simulink model "lfc_3area"  (R2026a)
settings: Solver=ode4  StopTime=60  FixedStep=0.01
model workspace (MATLAB code in the model file):
  | % lfc_params_3area.m
  | % ------------------------------------------------------------------------
  | % Parameters for the THREE-area LFC Simulink model (lfc_3area.slx).
  | %
  | % Physical parameters come from Table I of:
  | %   Shangguan et al., "Detection and Defense Against Multi-Point False Data
  | %   Injection Attacks of Load Frequency Control in Smart Grid,"
  | %   IEEE Trans. Smart Grid, vol. 16, no. 5, pp. 4143-4154, Sep. 2025.
  | %
  | % Each area's dual turbine-governor "a/b" entries are collapsed into a
  | % single-machine equivalent by averaging, so the per-area single-state
  | % equations (1a)-(1c) apply exactly (same convention as the Python
  | % replication in ../lfc_fdi_replication/config.py).
  | %
  | % Units: p.u. on a 3000 MVA base, frequency deviation in Hz.
  | % ------------------------------------------------------------------------
  | 
  | % ---- Area 1 ----
  | Tg1 = 0.320;  Tt1 = 0.065;  R1 = 2.835;  M1 = 0.1500;  D1 = 0.0640;
  | beta1 = 0.4250;  Kp1 = 0.0554;  Ki1 = 0.2285;
  | 
  | % ---- Area 2 ----
  | Tg2 = 0.305;  Tt2 = 0.080;  R2 = 2.945;  M2 = 0.1875;  D2 = 0.0964;
  | beta2 = 0.3966;  Kp2 = 0.0475;  Ki2 = 0.1764;
  | 
  | % ---- Area 3 ----
  | Tg3 = 0.320;  Tt3 = 0.060;  R3 = 2.725;  M3 = 0.1440;  D3 = 0.0850;
  | beta3 = 0.3552;  Kp3 = 0.0444;  Ki3 = 0.1866;
  | 
  | % ---- Tie-line synchronizing coefficients (Table I) ----
  | T12 = 0.243;  T13 = 0.321;  T23 = 0.195;
  | 
  | % ---- HVDC link equivalents per tie (average of the two areas' Kdc/Tdc) ----
  | % Area gains: Kdc = [0.90 1.10 0.86], Tdc = [0.50 0.55 0.48]
  | Kdc12 = 1.00;   Tdc12 = 0.525;
  | Kdc13 = 0.88;   Tdc13 = 0.490;
  | Kdc23 = 0.98;   Tdc23 = 0.515;
  | 
  | % ---- Nonlinearities (Section IV-A) ----
  | gdb = 6e-4;     % governor dead-band half-width [p.u.]
  | grc = 0.05;     % generation rate constraint [p.u./s]
  | 
  | % ---- Load / RES step disturbances per area ----
  | Pd1_t = 1;  Pd1_mag = 0.02;      % 0.02 p.u. load step in area 1 at t = 1 s
  | Pd2_t = 1;  Pd2_mag = 0;
  | Pd3_t = 1;  Pd3_mag = 0;
  | Pres1_t = 1;  Pres1_mag = 0;
  | Pres2_t = 1;  Pres2_mag = 0;
  | Pres3_t = 1;  Pres3_mag = 0;
  | 
  | % ---- FDI attack settings (Section II-B), one injector per channel -------
  | % Channel signal:  A(t) = gate(t) * [ step + samp*sin(w*(t-t0)) + pulse_train ]
  | % gate(t) = 1 for t0 <= t <= t1, else 0.  Set all magnitudes to 0 => no attack.
  | atk_pw = 3;                        % pulse on/off width [s]
  | chans = {'df1','df2','df3','pt1','pt2','pt3'};
  | for c = 1:numel(chans)
  |     ch = chans{c};
  |     eval(sprintf(['atk_%s_t0 = 20; atk_%s_t1 = 40; atk_%s_step = 0; ' ...
  |         'atk_%s_samp = 0; atk_%s_w = 2; atk_%s_pulse = 0;'], ...
  |         ch, ch, ch, ch, ch, ch));
  | end
  | clear chans c ch
undefined symbols (not defined in the file): atk_df1_pulse, atk_df1_samp, atk_df1_step, atk_df1_t0, atk_df1_t1, atk_df1_w, atk_df2_pulse, atk_df2_samp, atk_df2_step, atk_df2_t0, atk_df2_t1, atk_df2_w, atk_df3_pulse, atk_df3_samp, atk_df3_step, atk_df3_t0, atk_df3_t1, atk_df3_w, atk_pt1_pulse, atk_pt1_samp, atk_pt1_step, atk_pt1_t0, atk_pt1_t1, atk_pt1_w, atk_pt2_pulse, atk_pt2_samp, atk_pt2_step, atk_pt2_t0, atk_pt2_t1, atk_pt2_w, atk_pt3_pulse, atk_pt3_samp, atk_pt3_step, atk_pt3_t0, atk_pt3_t1, atk_pt3_w
settings Model: Creator=gunnalakistagoud  LastModifiedBy=gunnalakistagoud

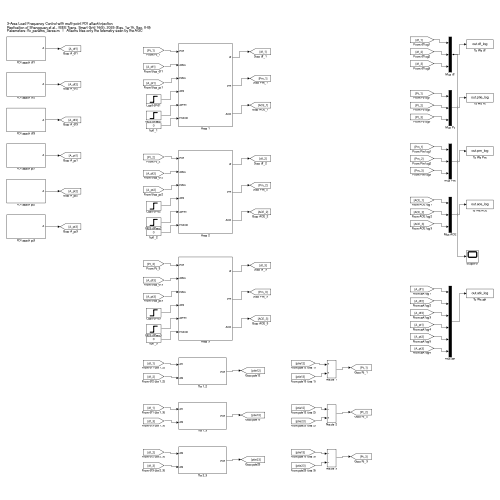
[thumbnail: Simulink's stored preview of the top-level diagram]
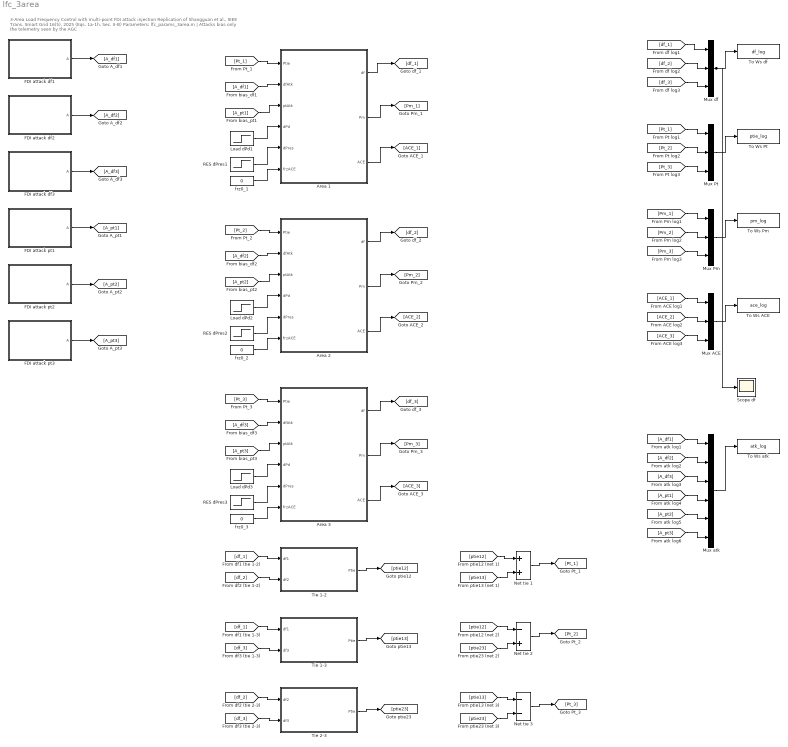
== system lfc_3area ==
  note: 3-Area Load Frequency Control with multi-point FDI attack injection
      | Replication of Shangguan et al., IEEE Trans. Smart Grid 16(5), 2025 (Eqs. 1a-1h, Sec. II-B)
      | Parameters: lfc_params_3area.m   |   Attacks bias only the telemetry seen by the AGC
  Area 1 : Subsystem
  Area 2 : Subsystem
  Area 3 : Subsystem
  FDI attack df1 : Subsystem
  FDI attack df2 : Subsystem
  FDI attack df3 : Subsystem
  FDI attack pt1 : Subsystem
  FDI attack pt2 : Subsystem
  FDI attack pt3 : Subsystem
  Load dPd1 : Step  Time=Pd1_t  FinalValue=Pd1_mag  SampleTime=0
  Load dPd2 : Step  Time=Pd2_t  FinalValue=Pd2_mag  SampleTime=0
  Load dPd3 : Step  Time=Pd3_t  FinalValue=Pd3_mag  SampleTime=0
  Mux ACE : Mux  Inputs=3
  Mux Pm : Mux  Inputs=3
  Mux Pt : Mux  Inputs=3
  Mux atk : Mux  Inputs=6
  Mux df : Mux  Inputs=3
  Net tie 1 : Sum
  Net tie 2 : Sum  Inputs=-+
  Net tie 3 : Sum  Inputs=--
  RES dPres1 : Step  Time=Pres1_t  FinalValue=Pres1_mag  SampleTime=0
  RES dPres2 : Step  Time=Pres2_t  FinalValue=Pres2_mag  SampleTime=0
  RES dPres3 : Step  Time=Pres3_t  FinalValue=Pres3_mag  SampleTime=0
  Scope df : Scope
  Tie 1-2 : Subsystem
  Tie 1-3 : Subsystem
  Tie 2-3 : Subsystem
  To Ws ACE : ToWorkspace  VariableName=ace_log  SaveFormat=Timeseries  SampleTime=-1
  To Ws Pm : ToWorkspace  VariableName=pm_log  SaveFormat=Timeseries  SampleTime=-1
  To Ws Pt : ToWorkspace  VariableName=ptie_log  SaveFormat=Timeseries  SampleTime=-1
  To Ws atk : ToWorkspace  VariableName=atk_log  SaveFormat=Timeseries  SampleTime=-1
  To Ws df : ToWorkspace  VariableName=df_log  SaveFormat=Timeseries  SampleTime=-1
  frz0_1 : Constant  Value=0
  frz0_2 : Constant  Value=0
  frz0_3 : Constant  Value=0
  wires:
  FDI attack df1/1(A) -> [A_df1]
  FDI attack df2/1(A) -> [A_df2]
  FDI attack df3/1(A) -> [A_df3]
  FDI attack pt1/1(A) -> [A_pt1]
  FDI attack pt2/1(A) -> [A_pt2]
  FDI attack pt3/1(A) -> [A_pt3]
  [Pt_1] -> Area 1/1(Ptie)
  [A_df1] -> Area 1/2(dfAtk)
  [A_pt1] -> Area 1/3(ptAtk)
  Load dPd1/1 -> Area 1/4(dPd)
  RES dPres1/1 -> Area 1/5(dPres)
  frz0_1/1 -> Area 1/6(frzACE)
  Area 1/1(df) -> [df_1]
  Area 1/2(Pm) -> [Pm_1]
  Area 1/3(ACE) -> [ACE_1]
  [Pt_2] -> Area 2/1(Ptie)
  [A_df2] -> Area 2/2(dfAtk)
  [A_pt2] -> Area 2/3(ptAtk)
  Load dPd2/1 -> Area 2/4(dPd)
  RES dPres2/1 -> Area 2/5(dPres)
  frz0_2/1 -> Area 2/6(frzACE)
  Area 2/1(df) -> [df_2]
  Area 2/2(Pm) -> [Pm_2]
  Area 2/3(ACE) -> [ACE_2]
  [Pt_3] -> Area 3/1(Ptie)
  [A_df3] -> Area 3/2(dfAtk)
  [A_pt3] -> Area 3/3(ptAtk)
  Load dPd3/1 -> Area 3/4(dPd)
  RES dPres3/1 -> Area 3/5(dPres)
  frz0_3/1 -> Area 3/6(frzACE)
  Area 3/1(df) -> [df_3]
  Area 3/2(Pm) -> [Pm_3]
  Area 3/3(ACE) -> [ACE_3]
  [df_1] -> Tie 1-2/1(df1)
  [df_2] -> Tie 1-2/2(df2)
  Tie 1-2/1(Ptie) -> [ptie12]
  [df_1] -> Tie 1-3/1(df1)
  [df_3] -> Tie 1-3/2(df3)
  Tie 1-3/1(Ptie) -> [ptie13]
  [df_2] -> Tie 2-3/1(df2)
  [df_3] -> Tie 2-3/2(df3)
  Tie 2-3/1(Ptie) -> [ptie23]
  [ptie12] -> Net tie 1/1
  [ptie13] -> Net tie 1/2
  Net tie 1/1 -> [Pt_1]
  [ptie12] -> Net tie 2/1
  [ptie23] -> Net tie 2/2
  Net tie 2/1 -> [Pt_2]
  [ptie13] -> Net tie 3/1
  [ptie23] -> Net tie 3/2
  Net tie 3/1 -> [Pt_3]
  [df_1] -> Mux df/1
  [df_2] -> Mux df/2
  [df_3] -> Mux df/3
  Mux df/1 -> To Ws df/1, Scope df/1
  [Pt_1] -> Mux Pt/1
  [Pt_2] -> Mux Pt/2
  [Pt_3] -> Mux Pt/3
  Mux Pt/1 -> To Ws Pt/1
  [Pm_1] -> Mux Pm/1
  [Pm_2] -> Mux Pm/2
  [Pm_3] -> Mux Pm/3
  Mux Pm/1 -> To Ws Pm/1
  [ACE_1] -> Mux ACE/1
  [ACE_2] -> Mux ACE/2
  [ACE_3] -> Mux ACE/3
  Mux ACE/1 -> To Ws ACE/1
  [A_df1] -> Mux atk/1
  [A_df2] -> Mux atk/2
  [A_df3] -> Mux atk/3
  [A_pt1] -> Mux atk/4
  [A_pt2] -> Mux atk/5
  [A_pt3] -> Mux atk/6
  Mux atk/1 -> To Ws atk/1

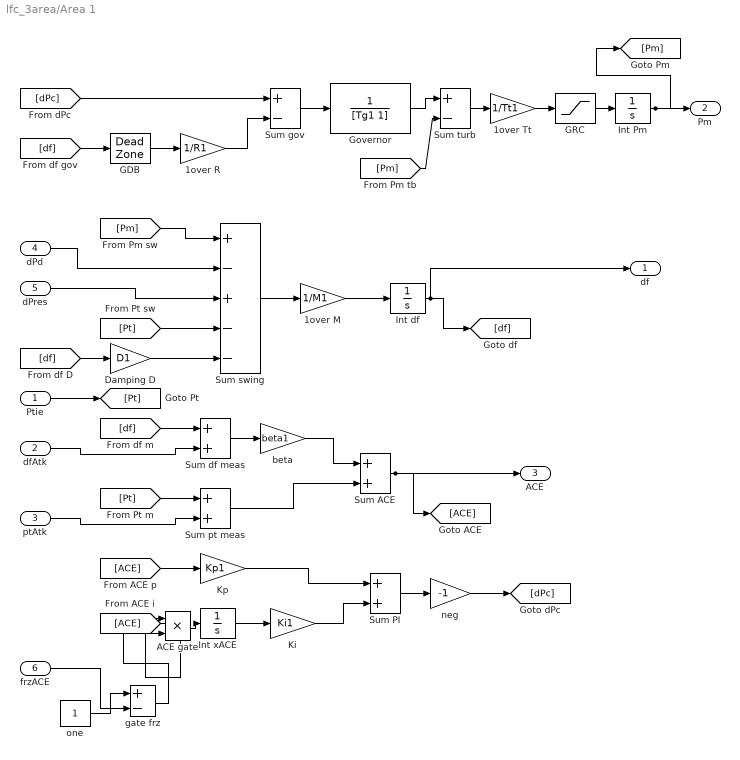
== system lfc_3area/Area 1 ==
  Ptie : Inport
  dfAtk : Inport  Port=2
  ptAtk : Inport  Port=3
  dPd : Inport  Port=4
  dPres : Inport  Port=5
  frzACE : Inport  Port=6
  1over M : Gain  Gain=1/M1
  1over R : Gain  Gain=1/R1
  1over Tt : Gain  Gain=1/Tt1
  ACE gate : Product
  Damping D : Gain  Gain=D1
  GDB : DeadZone  LowerValue=-gdb  UpperValue=gdb
  GRC : Saturate  UpperLimit=grc  LowerLimit=-grc
  Governor : TransferFcn  Denominator=[Tg1 1]
  Int Pm : Integrator
  Int df : Integrator
  Int xACE : Integrator
  Ki : Gain  Gain=Ki1
  Kp : Gain  Gain=Kp1
  Sum ACE : Sum
  Sum PI : Sum
  Sum df meas : Sum
  Sum gov : Sum  Inputs=+-
  Sum pt meas : Sum
  Sum swing : Sum  Inputs=+-+--
  Sum turb : Sum  Inputs=+-
  beta : Gain  Gain=beta1
  gate frz : Sum  Inputs=+-
  neg : Gain  Gain=-1
  one : Constant
  df : Outport
  Pm : Outport  Port=2
  ACE : Outport  Port=3
  wires:
  Ptie/1 -> [Pt]
  [Pm] -> Sum swing/1
  dPd/1 -> Sum swing/2
  dPres/1 -> Sum swing/3
  [Pt] -> Sum swing/4
  [df] -> Damping D/1
  Damping D/1 -> Sum swing/5
  Sum swing/1 -> 1over M/1
  1over M/1 -> Int df/1
  Int df/1 -> [df], df/1
  [df] -> GDB/1
  GDB/1 -> 1over R/1
  [dPc] -> Sum gov/1
  1over R/1 -> Sum gov/2
  Sum gov/1 -> Governor/1
  Governor/1 -> Sum turb/1
  [Pm] -> Sum turb/2
  Sum turb/1 -> 1over Tt/1
  1over Tt/1 -> GRC/1
  GRC/1 -> Int Pm/1
  Int Pm/1 -> [Pm], Pm/1
  [df] -> Sum df meas/1
  dfAtk/1 -> Sum df meas/2
  Sum df meas/1 -> beta/1
  [Pt] -> Sum pt meas/1
  ptAtk/1 -> Sum pt meas/2
  beta/1 -> Sum ACE/1
  Sum pt meas/1 -> Sum ACE/2
  Sum ACE/1 -> [ACE], ACE/1
  one/1 -> gate frz/1
  frzACE/1 -> gate frz/2
  [ACE] -> Kp/1
  [ACE] -> ACE gate/1
  gate frz/1 -> ACE gate/2
  ACE gate/1 -> Int xACE/1
  Int xACE/1 -> Ki/1
  Kp/1 -> Sum PI/1
  Ki/1 -> Sum PI/2
  Sum PI/1 -> neg/1
  neg/1 -> [dPc]

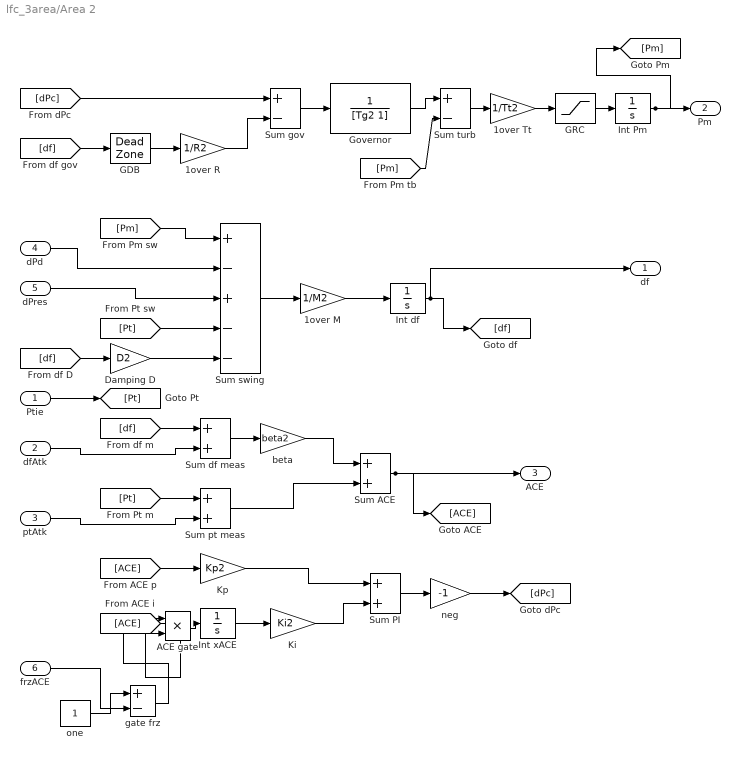
== system lfc_3area/Area 2 ==
  Ptie : Inport
  dfAtk : Inport  Port=2
  ptAtk : Inport  Port=3
  dPd : Inport  Port=4
  dPres : Inport  Port=5
  frzACE : Inport  Port=6
  1over M : Gain  Gain=1/M2
  1over R : Gain  Gain=1/R2
  1over Tt : Gain  Gain=1/Tt2
  ACE gate : Product
  Damping D : Gain  Gain=D2
  GDB : DeadZone  LowerValue=-gdb  UpperValue=gdb
  GRC : Saturate  UpperLimit=grc  LowerLimit=-grc
  Governor : TransferFcn  Denominator=[Tg2 1]
  Int Pm : Integrator
  Int df : Integrator
  Int xACE : Integrator
  Ki : Gain  Gain=Ki2
  Kp : Gain  Gain=Kp2
  Sum ACE : Sum
  Sum PI : Sum
  Sum df meas : Sum
  Sum gov : Sum  Inputs=+-
  Sum pt meas : Sum
  Sum swing : Sum  Inputs=+-+--
  Sum turb : Sum  Inputs=+-
  beta : Gain  Gain=beta2
  gate frz : Sum  Inputs=+-
  neg : Gain  Gain=-1
  one : Constant
  df : Outport
  Pm : Outport  Port=2
  ACE : Outport  Port=3
  wires:
  Ptie/1 -> [Pt]
  [Pm] -> Sum swing/1
  dPd/1 -> Sum swing/2
  dPres/1 -> Sum swing/3
  [Pt] -> Sum swing/4
  [df] -> Damping D/1
  Damping D/1 -> Sum swing/5
  Sum swing/1 -> 1over M/1
  1over M/1 -> Int df/1
  Int df/1 -> [df], df/1
  [df] -> GDB/1
  GDB/1 -> 1over R/1
  [dPc] -> Sum gov/1
  1over R/1 -> Sum gov/2
  Sum gov/1 -> Governor/1
  Governor/1 -> Sum turb/1
  [Pm] -> Sum turb/2
  Sum turb/1 -> 1over Tt/1
  1over Tt/1 -> GRC/1
  GRC/1 -> Int Pm/1
  Int Pm/1 -> [Pm], Pm/1
  [df] -> Sum df meas/1
  dfAtk/1 -> Sum df meas/2
  Sum df meas/1 -> beta/1
  [Pt] -> Sum pt meas/1
  ptAtk/1 -> Sum pt meas/2
  beta/1 -> Sum ACE/1
  Sum pt meas/1 -> Sum ACE/2
  Sum ACE/1 -> [ACE], ACE/1
  one/1 -> gate frz/1
  frzACE/1 -> gate frz/2
  [ACE] -> Kp/1
  [ACE] -> ACE gate/1
  gate frz/1 -> ACE gate/2
  ACE gate/1 -> Int xACE/1
  Int xACE/1 -> Ki/1
  Kp/1 -> Sum PI/1
  Ki/1 -> Sum PI/2
  Sum PI/1 -> neg/1
  neg/1 -> [dPc]

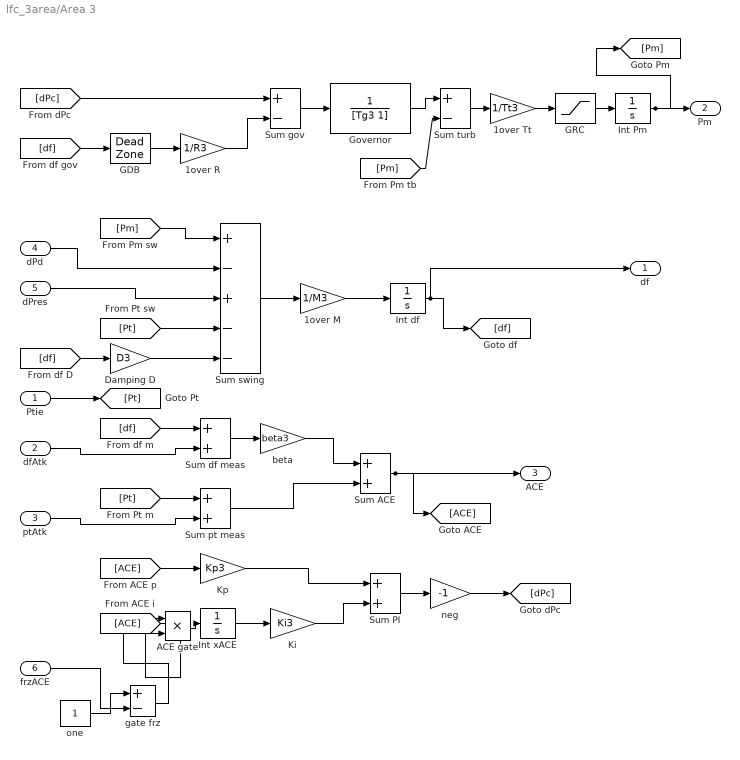
== system lfc_3area/Area 3 ==
  Ptie : Inport
  dfAtk : Inport  Port=2
  ptAtk : Inport  Port=3
  dPd : Inport  Port=4
  dPres : Inport  Port=5
  frzACE : Inport  Port=6
  1over M : Gain  Gain=1/M3
  1over R : Gain  Gain=1/R3
  1over Tt : Gain  Gain=1/Tt3
  ACE gate : Product
  Damping D : Gain  Gain=D3
  GDB : DeadZone  LowerValue=-gdb  UpperValue=gdb
  GRC : Saturate  UpperLimit=grc  LowerLimit=-grc
  Governor : TransferFcn  Denominator=[Tg3 1]
  Int Pm : Integrator
  Int df : Integrator
  Int xACE : Integrator
  Ki : Gain  Gain=Ki3
  Kp : Gain  Gain=Kp3
  Sum ACE : Sum
  Sum PI : Sum
  Sum df meas : Sum
  Sum gov : Sum  Inputs=+-
  Sum pt meas : Sum
  Sum swing : Sum  Inputs=+-+--
  Sum turb : Sum  Inputs=+-
  beta : Gain  Gain=beta3
  gate frz : Sum  Inputs=+-
  neg : Gain  Gain=-1
  one : Constant
  df : Outport
  Pm : Outport  Port=2
  ACE : Outport  Port=3
  wires:
  Ptie/1 -> [Pt]
  [Pm] -> Sum swing/1
  dPd/1 -> Sum swing/2
  dPres/1 -> Sum swing/3
  [Pt] -> Sum swing/4
  [df] -> Damping D/1
  Damping D/1 -> Sum swing/5
  Sum swing/1 -> 1over M/1
  1over M/1 -> Int df/1
  Int df/1 -> [df], df/1
  [df] -> GDB/1
  GDB/1 -> 1over R/1
  [dPc] -> Sum gov/1
  1over R/1 -> Sum gov/2
  Sum gov/1 -> Governor/1
  Governor/1 -> Sum turb/1
  [Pm] -> Sum turb/2
  Sum turb/1 -> 1over Tt/1
  1over Tt/1 -> GRC/1
  GRC/1 -> Int Pm/1
  Int Pm/1 -> [Pm], Pm/1
  [df] -> Sum df meas/1
  dfAtk/1 -> Sum df meas/2
  Sum df meas/1 -> beta/1
  [Pt] -> Sum pt meas/1
  ptAtk/1 -> Sum pt meas/2
  beta/1 -> Sum ACE/1
  Sum pt meas/1 -> Sum ACE/2
  Sum ACE/1 -> [ACE], ACE/1
  one/1 -> gate frz/1
  frzACE/1 -> gate frz/2
  [ACE] -> Kp/1
  [ACE] -> ACE gate/1
  gate frz/1 -> ACE gate/2
  ACE gate/1 -> Int xACE/1
  Int xACE/1 -> Ki/1
  Kp/1 -> Sum PI/1
  Ki/1 -> Sum PI/2
  Sum PI/1 -> neg/1
  neg/1 -> [dPc]

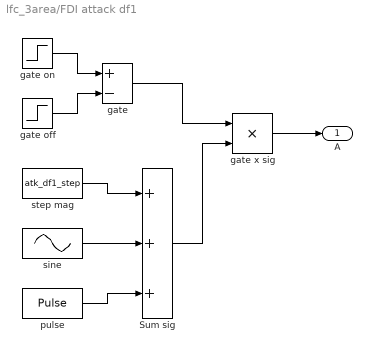
== system lfc_3area/FDI attack df1 ==
  Sum sig : Sum  Inputs=+++
  gate : Sum  Inputs=+-
  gate off : Step  Time=atk_df1_t1  SampleTime=0
  gate on : Step  Time=atk_df1_t0  SampleTime=0
  gate x sig : Product
  pulse : DiscretePulseGenerator  PulseType=Time based  Amplitude=atk_df1_pulse  Period=2*atk_pw  PulseWidth=50  PhaseDelay=atk_df1_t0
  sine : Sin  Amplitude=atk_df1_samp  Frequency=atk_df1_w  Phase=-atk_df1_w*atk_df1_t0  SampleTime=0
  step mag : Constant  Value=atk_df1_step
  A : Outport
  wires:
  gate on/1 -> gate/1
  gate off/1 -> gate/2
  step mag/1 -> Sum sig/1
  sine/1 -> Sum sig/2
  pulse/1 -> Sum sig/3
  gate/1 -> gate x sig/1
  Sum sig/1 -> gate x sig/2
  gate x sig/1 -> A/1

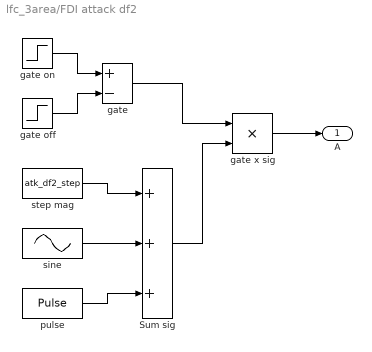
== system lfc_3area/FDI attack df2 ==
  Sum sig : Sum  Inputs=+++
  gate : Sum  Inputs=+-
  gate off : Step  Time=atk_df2_t1  SampleTime=0
  gate on : Step  Time=atk_df2_t0  SampleTime=0
  gate x sig : Product
  pulse : DiscretePulseGenerator  PulseType=Time based  Amplitude=atk_df2_pulse  Period=2*atk_pw  PulseWidth=50  PhaseDelay=atk_df2_t0
  sine : Sin  Amplitude=atk_df2_samp  Frequency=atk_df2_w  Phase=-atk_df2_w*atk_df2_t0  SampleTime=0
  step mag : Constant  Value=atk_df2_step
  A : Outport
  wires:
  gate on/1 -> gate/1
  gate off/1 -> gate/2
  step mag/1 -> Sum sig/1
  sine/1 -> Sum sig/2
  pulse/1 -> Sum sig/3
  gate/1 -> gate x sig/1
  Sum sig/1 -> gate x sig/2
  gate x sig/1 -> A/1

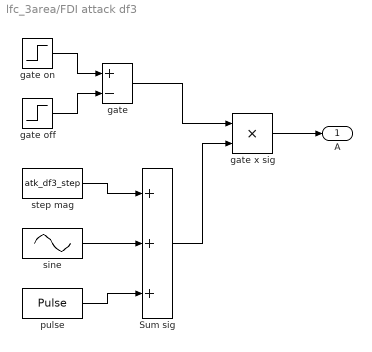
== system lfc_3area/FDI attack df3 ==
  Sum sig : Sum  Inputs=+++
  gate : Sum  Inputs=+-
  gate off : Step  Time=atk_df3_t1  SampleTime=0
  gate on : Step  Time=atk_df3_t0  SampleTime=0
  gate x sig : Product
  pulse : DiscretePulseGenerator  PulseType=Time based  Amplitude=atk_df3_pulse  Period=2*atk_pw  PulseWidth=50  PhaseDelay=atk_df3_t0
  sine : Sin  Amplitude=atk_df3_samp  Frequency=atk_df3_w  Phase=-atk_df3_w*atk_df3_t0  SampleTime=0
  step mag : Constant  Value=atk_df3_step
  A : Outport
  wires:
  gate on/1 -> gate/1
  gate off/1 -> gate/2
  step mag/1 -> Sum sig/1
  sine/1 -> Sum sig/2
  pulse/1 -> Sum sig/3
  gate/1 -> gate x sig/1
  Sum sig/1 -> gate x sig/2
  gate x sig/1 -> A/1

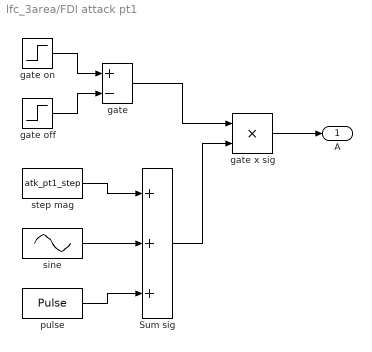
== system lfc_3area/FDI attack pt1 ==
  Sum sig : Sum  Inputs=+++
  gate : Sum  Inputs=+-
  gate off : Step  Time=atk_pt1_t1  SampleTime=0
  gate on : Step  Time=atk_pt1_t0  SampleTime=0
  gate x sig : Product
  pulse : DiscretePulseGenerator  PulseType=Time based  Amplitude=atk_pt1_pulse  Period=2*atk_pw  PulseWidth=50  PhaseDelay=atk_pt1_t0
  sine : Sin  Amplitude=atk_pt1_samp  Frequency=atk_pt1_w  Phase=-atk_pt1_w*atk_pt1_t0  SampleTime=0
  step mag : Constant  Value=atk_pt1_step
  A : Outport
  wires:
  gate on/1 -> gate/1
  gate off/1 -> gate/2
  step mag/1 -> Sum sig/1
  sine/1 -> Sum sig/2
  pulse/1 -> Sum sig/3
  gate/1 -> gate x sig/1
  Sum sig/1 -> gate x sig/2
  gate x sig/1 -> A/1

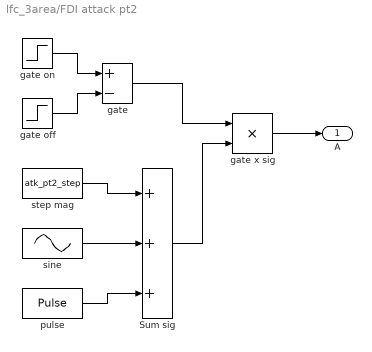
== system lfc_3area/FDI attack pt2 ==
  Sum sig : Sum  Inputs=+++
  gate : Sum  Inputs=+-
  gate off : Step  Time=atk_pt2_t1  SampleTime=0
  gate on : Step  Time=atk_pt2_t0  SampleTime=0
  gate x sig : Product
  pulse : DiscretePulseGenerator  PulseType=Time based  Amplitude=atk_pt2_pulse  Period=2*atk_pw  PulseWidth=50  PhaseDelay=atk_pt2_t0
  sine : Sin  Amplitude=atk_pt2_samp  Frequency=atk_pt2_w  Phase=-atk_pt2_w*atk_pt2_t0  SampleTime=0
  step mag : Constant  Value=atk_pt2_step
  A : Outport
  wires:
  gate on/1 -> gate/1
  gate off/1 -> gate/2
  step mag/1 -> Sum sig/1
  sine/1 -> Sum sig/2
  pulse/1 -> Sum sig/3
  gate/1 -> gate x sig/1
  Sum sig/1 -> gate x sig/2
  gate x sig/1 -> A/1

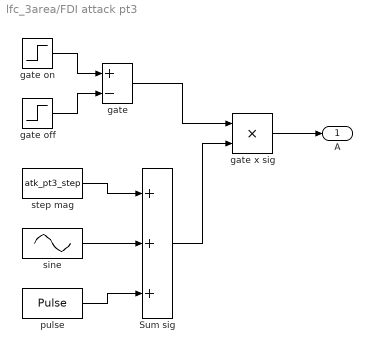
== system lfc_3area/FDI attack pt3 ==
  Sum sig : Sum  Inputs=+++
  gate : Sum  Inputs=+-
  gate off : Step  Time=atk_pt3_t1  SampleTime=0
  gate on : Step  Time=atk_pt3_t0  SampleTime=0
  gate x sig : Product
  pulse : DiscretePulseGenerator  PulseType=Time based  Amplitude=atk_pt3_pulse  Period=2*atk_pw  PulseWidth=50  PhaseDelay=atk_pt3_t0
  sine : Sin  Amplitude=atk_pt3_samp  Frequency=atk_pt3_w  Phase=-atk_pt3_w*atk_pt3_t0  SampleTime=0
  step mag : Constant  Value=atk_pt3_step
  A : Outport
  wires:
  gate on/1 -> gate/1
  gate off/1 -> gate/2
  step mag/1 -> Sum sig/1
  sine/1 -> Sum sig/2
  pulse/1 -> Sum sig/3
  gate/1 -> gate x sig/1
  Sum sig/1 -> gate x sig/2
  gate x sig/1 -> A/1

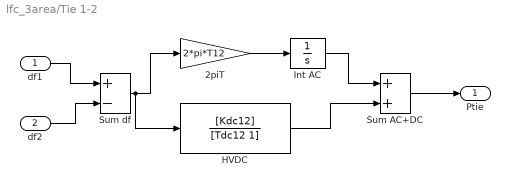
== system lfc_3area/Tie 1-2 ==
  df1 : Inport
  df2 : Inport  Port=2
  2piT : Gain  Gain=2*pi*T12
  HVDC : TransferFcn  Numerator=[Kdc12]  Denominator=[Tdc12 1]
  Int AC : Integrator
  Sum AC+DC : Sum
  Sum df : Sum  Inputs=+-
  Ptie : Outport
  wires:
  df1/1 -> Sum df/1
  df2/1 -> Sum df/2
  Sum df/1 -> 2piT/1, HVDC/1
  2piT/1 -> Int AC/1
  Int AC/1 -> Sum AC+DC/1
  HVDC/1 -> Sum AC+DC/2
  Sum AC+DC/1 -> Ptie/1

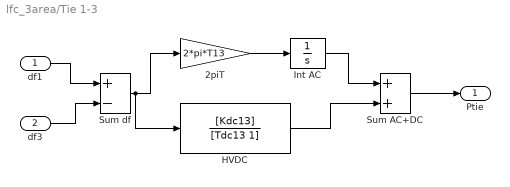
== system lfc_3area/Tie 1-3 ==
  df1 : Inport
  df3 : Inport  Port=2
  2piT : Gain  Gain=2*pi*T13
  HVDC : TransferFcn  Numerator=[Kdc13]  Denominator=[Tdc13 1]
  Int AC : Integrator
  Sum AC+DC : Sum
  Sum df : Sum  Inputs=+-
  Ptie : Outport
  wires:
  df1/1 -> Sum df/1
  df3/1 -> Sum df/2
  Sum df/1 -> 2piT/1, HVDC/1
  2piT/1 -> Int AC/1
  Int AC/1 -> Sum AC+DC/1
  HVDC/1 -> Sum AC+DC/2
  Sum AC+DC/1 -> Ptie/1

== system lfc_3area/Tie 2-3 ==
  df2 : Inport
  df3 : Inport  Port=2
  2piT : Gain  Gain=2*pi*T23
  HVDC : TransferFcn  Numerator=[Kdc23]  Denominator=[Tdc23 1]
  Int AC : Integrator
  Sum AC+DC : Sum
  Sum df : Sum  Inputs=+-
  Ptie : Outport
  wires:
  df2/1 -> Sum df/1
  df3/1 -> Sum df/2
  Sum df/1 -> 2piT/1, HVDC/1
  2piT/1 -> Int AC/1
  Int AC/1 -> Sum AC+DC/1
  HVDC/1 -> Sum AC+DC/2
  Sum AC+DC/1 -> Ptie/1
